simulink model "scon2_L9_1ponto3_simulink"  (R2024a)
settings: Solver=VariableStepAuto  StartTime=0.0  StopTime=10.0  RelTol=1e-3
values from neighbouring files (symbols this model uses):
  A = [0, 1; -7, -2]    [scon2_L9_1ponto3.m]
  B = [0; 1]    [scon2_L9_1ponto3.m]
  C = [1, 4]    [scon2_L9_1ponto3.m]
  K = acker(A, B, J_c)    [scon2_L9_1ponto3.m]
  K_e = acker(A', C', J_o)'    [scon2_L9_1ponto3.m]
  x0 = [0; 0]    [scon2_L9_1ponto3.m]
settings Model: Creator=Carlos Augusto  LastModifiedBy=Carlos Augusto

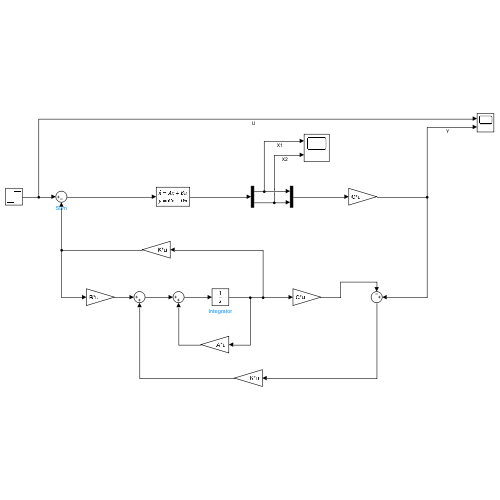
[thumbnail: Simulink's stored preview of the top-level diagram]
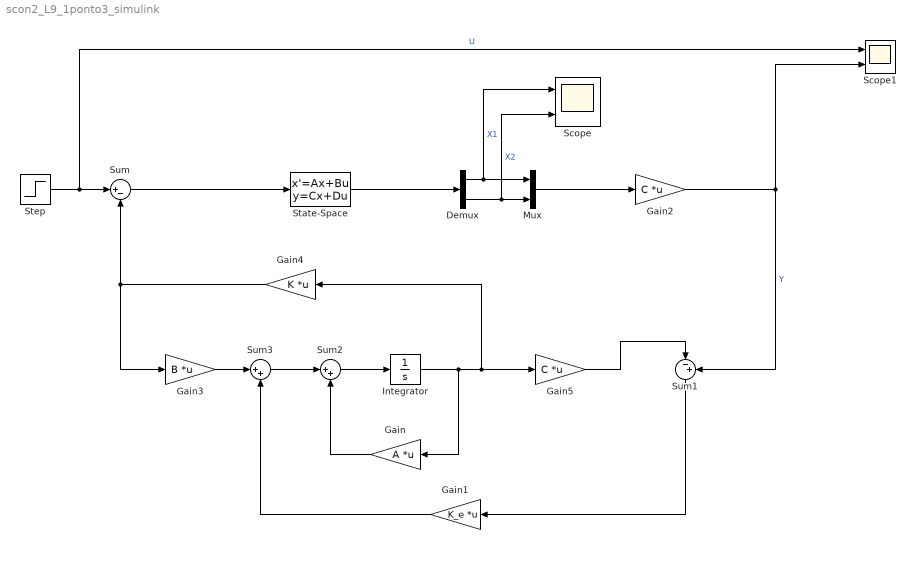
== system scon2_L9_1ponto3_simulink ==
  Demux : Demux  Outputs=2
  Gain : Gain  Gain=A  Multiplication=Matrix(K*u)
  Gain1 : Gain  Gain=K_e  Multiplication=Matrix(K*u)
  Gain2 : Gain  Gain=C  Multiplication=Matrix(K*u)
  Gain3 : Gain  Gain=B  Multiplication=Matrix(K*u)
  Gain4 : Gain  Gain=K  Multiplication=Matrix(K*u)
  Gain5 : Gain  Gain=C  Multiplication=Matrix(K*u)
  Integrator : Integrator
  Mux : Mux  Inputs=2
  Scope : Scope  NumInputPorts=2
  Scope1 : Scope  NumInputPorts=2
  State-Space : StateSpace  A=A  B=B  C=eye(2)  D=zeros(2,1)  InitialCondition=x0
  Step : Step  SampleTime=0
  Sum : Sum  Inputs=|+-
  Sum1 : Sum  Inputs=|-+
  Sum2 : Sum  Inputs=|++
  Sum3 : Sum  Inputs=|++
  wires:
  State-Space/1 -> Demux/1
  Demux/1 -> Mux/1, Scope/1  "X1"
  Demux/2 -> Mux/2, Scope/2  "X2"
  Step/1 -> Sum/1, Scope1/1  "U"
  Sum/1 -> State-Space/1
  Mux/1 -> Gain2/1
  Gain4/1 -> Gain3/1, Sum/2
  Gain2/1 -> Sum1/2, Scope1/2  "Y"
  Gain5/1 -> Sum1/1
  Integrator/1 -> Gain/1, Gain5/1, Gain4/1
  Sum1/1 -> Gain1/1
  Sum2/1 -> Integrator/1
  Sum3/1 -> Sum2/1
  Gain3/1 -> Sum3/1
  Gain1/1 -> Sum3/2
  Gain/1 -> Sum2/2
